simulink model "FixedWing_Dynamic_Model_SIL_simulink_PX4"  (R2023a)
settings: Solver=ode4  StartTime=0.0  StopTime=130  FixedStep=0.004  RelTol=1e-3
model workspace (MAT data in the model file):
  sample_time = 0.004
values from neighbouring files (symbols this model uses):
  env = struct    [InitEnvironment.m]
  frecuency = 0.012    [PX4_var_controllers.m]
  g = 9.81    [PX4_var_controllers.m]
  home_alt = 171    [InitSimulinkPlantVars.m]    (also in PX4_var_controllers.m)
  home_lat = 39.49738807491014    (= 39.4973880749)    [InitSimulinkPlantVars.m]    (also in PX4_var_controllers.m)
  home_lon = -0.6268122488722822    (= -0.626812248872)    [InitSimulinkPlantVars.m]    (also in PX4_var_controllers.m)
  mission = [wp]    [PX4_var_controllers.m]
  nwap = 9    [PX4_var_controllers.m]
  pitch_D = 0    [PX4_var_controllers.m]
  pitch_ff = 0.4    [PX4_var_controllers.m]
  pitch_I = 0.05    [PX4_var_controllers.m]
  pitch_P = 0.05    [PX4_var_controllers.m]
  poswp = [poswp1;poswp2;poswp3;poswp4;poswp5;poswp6;poswp7;poswp8;poswp9]    [PX4_var_controllers.m]
  roll_D = 0    [PX4_var_controllers.m]
  roll_ff = 0.4    [PX4_var_controllers.m]
  roll_I = 0.13    [PX4_var_controllers.m]
  roll_P = 0.085    [PX4_var_controllers.m]
  tc_pitch = 0.4    [PX4_var_controllers.m]
  tc_roll = 0.45    [PX4_var_controllers.m]
  uavData = struct    [InitFixedWingParam.m]
  V_cruise = [15,15,15,20,25,25,20,15,15]    [PX4_var_controllers.m]
  yaw_D = 0    [PX4_var_controllers.m]
  yaw_ff = 0.3    [PX4_var_controllers.m]
  yaw_I = 0.1    [PX4_var_controllers.m]
  yaw_P = 0.05    [PX4_var_controllers.m]
undefined symbols (not defined in the file or in its folder): DiscIntNeverNeededParam, Earth, LC, TEBCL, TECL, TECS, WGS84
libraries: aerolibactuator x5, aerolibasang x4, slpidlib x3, uavalgslib x2, aerolibatmos2 x2, shared6dof x1, aerolibtransform2 x1, aerolibconvert2 x1, simulink_extras x1
(part 3 of 3)

== system FixedWing_Dynamic_Model_SIL_simulink_PX4/Dynamics/Fixed-wing UAV Dynamics/Force and Moment Calculation/Aerodynamic Forces and Moments/Compute Body Frame Forces and Moments/Wind frame F& M/Lateral Channel/Cl/roll factors/roll rate fact ==
  p : Inport
  Airspeed : Inport  Port=2
  Cmq1 : Constant  Value=.5
      settings: AttributesFormatString=%<Value>
  Cmq2 : Constant  Value=uavData.geometry.span
      settings: AttributesFormatString=%<Value>
  Product : Product  Inputs=***/  SaturateOnIntegerOverflow=on  OutDataTypeStr=Inherit: Same as first input
  Saturation : Saturate  UpperLimit=inf  LowerLimit=0.1
      settings: AttributesFormatString="[%<LowerLimit>  %<UpperLimit>]"
  Roll Rate Fac : Outport  VectorParamsAs1DForOutWhenUnconnected=off
  wires:
  Saturation/1 -> Product/4
  Airspeed/1 -> Saturation/1
  Cmq2/1 -> Product/3
  Cmq1/1 -> Product/2
  p/1 -> Product/1
  Product/1 -> Roll Rate Fac/1

== system FixedWing_Dynamic_Model_SIL_simulink_PX4/Dynamics/Fixed-wing UAV Dynamics/Force and Moment Calculation/Aerodynamic Forces and Moments/Compute Body Frame Forces and Moments/Wind frame F& M/Lateral Channel/Cl/roll factors/yaw rate fact ==
  r : Inport
  Airspeed : Inport  Port=2
  Cmq3 : Constant  Value=.5
      settings: AttributesFormatString=%<Value>
  Cmq4 : Constant  Value=uavData.geometry.span
      settings: AttributesFormatString=%<Value>
  Product1 : Product  Inputs=***/  SaturateOnIntegerOverflow=on  OutDataTypeStr=Inherit: Same as first input
  Saturation : Saturate  UpperLimit=inf  LowerLimit=0.1
      settings: AttributesFormatString="[%<LowerLimit>  %<UpperLimit>]"
  Yaw Rate Fac : Outport  VectorParamsAs1DForOutWhenUnconnected=off
  wires:
  Product1/1 -> Yaw Rate Fac/1
  r/1 -> Product1/1
  Cmq3/1 -> Product1/2
  Cmq4/1 -> Product1/3
  Airspeed/1 -> Saturation/1
  Saturation/1 -> Product1/4

== system FixedWing_Dynamic_Model_SIL_simulink_PX4/Dynamics/Fixed-wing UAV Dynamics/Force and Moment Calculation/Aerodynamic Forces and Moments/Compute Body Frame Forces and Moments/Wind frame F& M/Lateral Channel/Cn/yaw factors/roll rate fact ==
  p : Inport
  Airspeed : Inport  Port=2
  Cmq1 : Constant  Value=.5
      settings: AttributesFormatString=%<Value>
  Cmq2 : Constant  Value=uavData.geometry.span
      settings: AttributesFormatString=%<Value>
  Product : Product  Inputs=***/  SaturateOnIntegerOverflow=on  OutDataTypeStr=Inherit: Same as first input
  Saturation : Saturate  UpperLimit=inf  LowerLimit=0.1
      settings: AttributesFormatString="[%<LowerLimit>  %<UpperLimit>]"
  Roll Rate Fac : Outport  VectorParamsAs1DForOutWhenUnconnected=off
  wires:
  Saturation/1 -> Product/4
  Airspeed/1 -> Saturation/1
  Cmq2/1 -> Product/3
  Cmq1/1 -> Product/2
  p/1 -> Product/1
  Product/1 -> Roll Rate Fac/1

== system FixedWing_Dynamic_Model_SIL_simulink_PX4/Dynamics/Fixed-wing UAV Dynamics/Force and Moment Calculation/Aerodynamic Forces and Moments/Compute Body Frame Forces and Moments/Wind frame F& M/Lateral Channel/Cn/yaw factors/yaw rate fact ==
  r : Inport
  Airspeed : Inport  Port=2
  Cmq3 : Constant  Value=.5
      settings: AttributesFormatString=%<Value>
  Cmq4 : Constant  Value=uavData.geometry.span
      settings: AttributesFormatString=%<Value>
  Product1 : Product  Inputs=***/  SaturateOnIntegerOverflow=on  OutDataTypeStr=Inherit: Same as first input
  Saturation : Saturate  UpperLimit=inf  LowerLimit=0.1
      settings: AttributesFormatString="[%<LowerLimit>  %<UpperLimit>]"
  Yaw Rate Fac : Outport  VectorParamsAs1DForOutWhenUnconnected=off
  wires:
  Product1/1 -> Yaw Rate Fac/1
  r/1 -> Product1/1
  Cmq3/1 -> Product1/2
  Cmq4/1 -> Product1/3
  Airspeed/1 -> Saturation/1
  Saturation/1 -> Product1/4

== system FixedWing_Dynamic_Model_SIL_simulink_PX4/Dynamics/Fixed-wing UAV Dynamics/Force and Moment Calculation/Aerodynamic Forces and Moments/Compute Body Frame Forces and Moments/Wind frame F& M/Longitudinal Channel/CL/Lift due to pitch rate/pitch rate factor ==
  q : Inport
  Airspeed : Inport  Port=2
  Cmq2 : Constant  Value=uavData.geometry.chord
      settings: AttributesFormatString=%<Value>
  Product : Product  Inputs=**/  SaturateOnIntegerOverflow=on  OutDataTypeStr=Inherit: Same as first input
  Saturation : Saturate  UpperLimit=inf  LowerLimit=0.1
      settings: AttributesFormatString="[%<LowerLimit>  %<UpperLimit>]"
  Pitch Rate Fac : Outport  VectorParamsAs1DForOutWhenUnconnected=off
  wires:
  Saturation/1 -> Product/3
  Cmq2/1 -> Product/2
  Airspeed/1 -> Saturation/1
  q/1 -> Product/1
  Product/1 -> Pitch Rate Fac/1

== matlab function FixedWing_Dynamic_Model_SIL_simulink_PX4/Controllers/Total Energy control system/Total energy balance control loop/MATLAB Function1 ==
  data: SEB_rate_correction input; pitch_setpoint_1 output; V_TAS input
function pitch_setpoint_1  = seb_to_pitch(SEB_rate_correction,V_TAS)

g = 9.81;
airspeed_for_seb_rate = 15;

if V_TAS > 10^-6

airspeed_for_seb_rate = V_TAS;
end 

climb_angle_to_SEB_rate = airspeed_for_seb_rate*g;

pitch_setpoint_1 = SEB_rate_correction/climb_angle_to_SEB_rate;

== matlab function FixedWing_Dynamic_Model_SIL_simulink_PX4/Controllers/L1 Controller/MATLAB Function1 ==
  data: eta input; eta output
function eta = fcn(eta)
eta = mod(eta,2*pi);
if eta>pi
    eta = eta-2*pi;
end

== matlab function FixedWing_Dynamic_Model_SIL_simulink_PX4/Controllers/Attitude Controller/MATLAB Function2 ==
  data: roll_setpoint input; roll_body_rate_setpoint_raw output; roll input; euler_yaw_rate_setpoint input; tc input; pitch input
function roll_body_rate_setpoint_raw = roll_crtl(roll_setpoint,roll,euler_yaw_rate_setpoint,tc,pitch)
roll_error = roll_setpoint-roll;
euler_rate_setpoint = roll_error /tc;
roll_body_rate_setpoint_raw = euler_rate_setpoint - sin(pitch)*euler_yaw_rate_setpoint;

== matlab function FixedWing_Dynamic_Model_SIL_simulink_PX4/Controllers/Attitude Controller/MATLAB Function3 ==
  data: pitch_body_rate_setpoint_raw output; pitch input; euler_yaw_rate_setpoint input; roll input; euler_rate_setpoint_pitch input
function pitch_body_rate_setpoint_raw  = pitch_crtl(pitch,euler_yaw_rate_setpoint,roll,euler_rate_setpoint_pitch)

pitch_body_rate_setpoint_raw = cos(roll)*euler_rate_setpoint_pitch+cos(pitch)*sin(roll)*euler_yaw_rate_setpoint;

== matlab function FixedWing_Dynamic_Model_SIL_simulink_PX4/Controllers/Attitude Controller/MATLAB Function4 ==
  data: roll input; yaw_body_rate_setpoint_raw output; pitch input; euler_pitch_rate_setpoint input; euler_rate_setpoint_yaw input
function yaw_body_rate_setpoint_raw    = yaw_crtl(roll,pitch,euler_pitch_rate_setpoint,euler_rate_setpoint_yaw)

yaw_body_rate_setpoint_raw = -sin(roll)*euler_pitch_rate_setpoint+cos(roll)*cos(pitch)*euler_rate_setpoint_yaw;

== matlab function FixedWing_Dynamic_Model_SIL_simulink_PX4/Controllers/MATLAB Function1 ==
  data: tas_error_percentage input; ratio_undersped output; equivalent_airspeed_trim input; tas_min input; tas input
function ratio_undersped = ratio_underspeed(tas_error_percentage,equivalent_airspeed_trim,tas_min,tas)

tas_error_bound = tas_error_percentage*equivalent_airspeed_trim;
tas_undersped_soft_bound = tas_error_bound*equivalent_airspeed_trim;

tas_fully_undersped = max(tas_min-tas_error_bound-tas_undersped_soft_bound,0);
tas_starting_to_undersped = max(tas_min-tas_error_bound,tas_fully_undersped);

ratio_undersped = 1-((norm(tas)-tas_fully_undersped)/max(tas_starting_to_undersped-tas_fully_undersped,10^-6));

== matlab function FixedWing_Dynamic_Model_SIL_simulink_PX4/Controllers/Attitude Controller/MATLAB Function5 ==
  data: roll input; euler_rate_setpoint_yaw output; euler_rate_setpoint_pitch output; roll_setpoint input; pitch input; airspeed input; pitch_setpoint input; tc input
function [euler_rate_setpoint_yaw,euler_rate_setpoint_pitch] = euler_rate(roll,roll_setpoint,pitch,airspeed,pitch_setpoint,tc)
g = 9.81;
contrained_roll = min(max(roll,-abs(roll_setpoint)),abs(roll_setpoint));
euler_rate_setpoint_yaw = tan(contrained_roll)*cos(pitch)*g/airspeed; % turn coordination

pitch_error = pitch_setpoint-pitch;
euler_rate_setpoint_pitch = pitch_error/tc;

== matlab function FixedWing_Dynamic_Model_SIL_simulink_PX4/Controllers/Total Energy control system/Total energy control loop/MATLAB Function4 ==
  data: throttle_max input; throttle_min input; throttle_integ_input input; throttle_integ_state output
function throttle_integ_state = T_integ(throttle_max,throttle_min, throttle_integ_input)

if throttle_integ_input >= throttle_max
    throttle_integ_input = min(0,throttle_integ_input);
elseif throttle_integ_input<= throttle_min
    throttle_integ_input = max(0,throttle_integ_input);
end
    throttle_integ_state = throttle_integ_input;

== matlab function FixedWing_Dynamic_Model_SIL_simulink_PX4/Controllers/Total Energy control system/Total energy balance control loop/MATLAB Function4 ==
  data: vert_accel_limit input; pitch_increment output; V_TAS input
function pitch_increment = pitch_incre(vert_accel_limit,V_TAS)

pitch_increment = vert_accel_limit / max(V_TAS,10^-6);

== matlab function FixedWing_Dynamic_Model_SIL_simulink_PX4/Controllers/Total Energy control system/Total energy balance control loop/MATLAB Function5 ==
  data: pitch_setpoint input; pitch_increment input; pitch_setpoint output
function pitch_setpoint = pitch_incre_lim(pitch_setpoint,pitch_increment)
pitch_setpoint = min(max(pitch_setpoint,pitch_setpoint-pitch_increment),pitch_setpoint+pitch_increment);

== matlab function FixedWing_Dynamic_Model_SIL_simulink_PX4/Controllers/MATLAB Function4 ==
  data: ratio_undersped input; weight_spe output; pitch_speed_weight input; weight_ske output
function [weight_spe,weight_ske] = weight(ratio_undersped,pitch_speed_weight)

pitch_speed_weight = min(max(pitch_speed_weight,0),2);

if ratio_undersped>10^-6
    pitch_speed_weight = 2*ratio_undersped+(1-ratio_undersped)*pitch_speed_weight;
end

weight_spe = min(max(2-pitch_speed_weight,0),1);
weight_ske = min(max(pitch_speed_weight,0),1);

== matlab function FixedWing_Dynamic_Model_SIL_simulink_PX4/Controllers/Total Energy control system/Total energy control loop/MATLAB Function2 ==
  data: ste_rate input; ste_rate_max input; T_FF output; ste_rate_min input; throttle_max input; throttle_min input; throttle_trim input
function T_FF  = T_predicted(ste_rate,ste_rate_max, ste_rate_min, throttle_max, throttle_min, throttle_trim)
throttle_above_trim_per_ste_rate = (throttle_max - throttle_trim)/ste_rate_max;
throttle_below_trim_per_ste_rate = (throttle_trim - throttle_min)/ste_rate_min;

if ste_rate >= 10^-6
    T_FF = throttle_trim + ste_rate*throttle_above_trim_per_ste_rate;
else
    T_FF = throttle_trim - ste_rate*throttle_below_trim_per_ste_rate;
end

== matlab function FixedWing_Dynamic_Model_SIL_simulink_PX4/Controllers/Total Energy control system/Total energy balance control loop/MATLAB Function2 ==
  data: SEB_rate_correction input; pitch_setpoint_1 output; V_TAS input
function pitch_setpoint_1  = seb_to_pitch(SEB_rate_correction,V_TAS)

g = 9.81;
airspeed_for_seb_rate = 15;

if V_TAS > 10^-6

airspeed_for_seb_rate = V_TAS;
end 

climb_angle_to_SEB_rate = airspeed_for_seb_rate*g;

pitch_setpoint_1 = SEB_rate_correction/climb_angle_to_SEB_rate;

== matlab function FixedWing_Dynamic_Model_SIL_simulink_PX4/Controllers/Seguimiento waypoints/MATLAB Function4 ==
  data: Vcruise input; velocidad output; current_wp input; poswp input; nwap input
function velocidad  = vel(Vcruise, current_wp,poswp,nwap)

velocidad = Vcruise(1);
for i = 1:nwap
    if current_wp(1) == poswp(i,1)
        velocidad = Vcruise(i);
    end
end

== matlab function FixedWing_Dynamic_Model_SIL_simulink_PX4/Controllers/MATLAB Function ==
  data: vxyz input; course output; gndspeed output
function [course, gndspeed] = cour_gnds(vxyz)

vx = vxyz(1);
vy = vxyz(2);

course = atan2(vy,vx);
gndspeed = norm([vx,vy]);

== matlab function FixedWing_Dynamic_Model_SIL_simulink_PX4/Controllers/Total Energy control system/Total energy balance control loop/MATLAB Function3 ==
  data: pitch_max input; pitch_integ_state output; pitch_min input; pitch_integ_input input
function pitch_integ_state = p_integ(pitch_max,pitch_min,pitch_integ_input)
if pitch_integ_input >= pitch_max
    pitch_integ_input = min(pitch_integ_input,0);
elseif pitch_integ_input <= pitch_min
    pitch_integ_input = max(pitch_integ_input,0);
end
pitch_integ_state = pitch_integ_input;

== matlab function FixedWing_Dynamic_Model_SIL_simulink_PX4/Controllers/Seguimiento waypoints/MATLAB Function2 ==
  data: toWP input; wps output; fromWP input; alt output
function [wps, alt]= waypoints_alt(toWP, fromWP)
    wps = zeros(2,3); 
    wps = [fromWP'; toWP'];
    alt = -toWP(3);
end

== matlab function FixedWing_Dynamic_Model_SIL_simulink_PX4/Controllers/MATLAB Function2 ==
  data: max_climb_rate input; ste_rate_to_throttle output; min_sink_rate input; ste_rate_max output; ste_rate_min output
function [ste_rate_to_throttle,ste_rate_max,ste_rate_min]  = ste(max_climb_rate,min_sink_rate)
 g = 9.81;
ste_rate_max = max(max_climb_rate,10^-6)*g;
ste_rate_min = -max(min_sink_rate,10^-6)*g;

ste_rate_to_throttle = 1/(ste_rate_max-ste_rate_min);

== matlab function FixedWing_Dynamic_Model_SIL_simulink_PX4/Controllers/MATLAB Function3 ==
  data: ste_rate_max input; airspeed_rate_output output; ste_rate_min input; V_TAS input; airspeed_rate input
function airspeed_rate_output = V_rate(ste_rate_max,ste_rate_min,V_TAS,airspeed_rate)
max_tas_rate_sp = 0.5*ste_rate_max/max(V_TAS,10^-6);
min_tas_rate_sp = 0.5*ste_rate_min/max(V_TAS,10^-6);

airspeed_rate_output = min(max(airspeed_rate,min_tas_rate_sp),max_tas_rate_sp);
